simulink model "MPC_P2_2026_1"  (R2024b)
settings: Solver=VariableStepAuto  StartTime=0.0  StopTime=20  RelTol=1e-3
settings Model: Creator=Asus  LastModifiedBy=CARLOS
settings ModelReferenceCC: UpdateModelReferenceTargets=IfOutOfDate

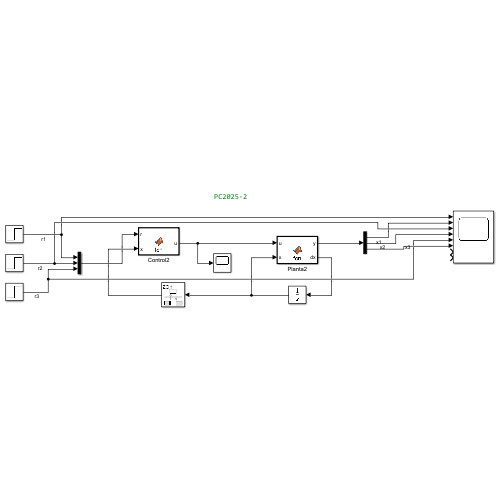
[thumbnail: Simulink's stored preview of the top-level diagram]
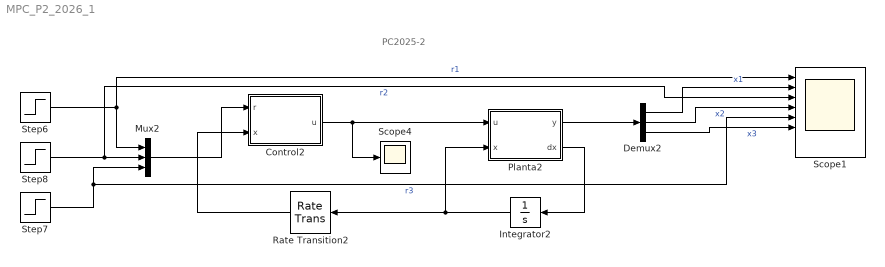
== system MPC_P2_2026_1 ==
  note: PC2025-2
  Control2 : MATLAB Function  TreatAsAtomicUnit=on
  Demux2 : Demux  Outputs=3
  Integrator2 : Integrator  InitialCondition=[0; 0; 0]
  Mux2 : Mux  Inputs=3
  Planta2 : MATLAB Function  TreatAsAtomicUnit=on
  Rate Transition2 : RateTransition  OutPortSampleTime=T
  Scope1 : Scope  NumInputPorts=8
  Scope4 : Scope
  Step6 : Step  After=0  SampleTime=0
  Step7 : Step  SampleTime=0
  Step8 : Step  After=0  SampleTime=0
  wires:
  Rate Transition2/1 -> Control2/2(x)
  Integrator2/1 -> Planta2/2(x), Rate Transition2/1
  Demux2/1 -> Scope1/2  "x1"
  Demux2/3 -> Scope1/6  "x3"
  Demux2/2 -> Scope1/4  "x2"
  Step7/1 -> Scope1/5, Mux2/3  "r3"
  Step8/1 -> Scope1/3, Mux2/2  "r2"
  Planta2/1(y) -> Demux2/1
  Step6/1 -> Mux2/1, Scope1/1  "r1"
  Control2/1(u) -> Scope4/1, Planta2/1(u)
  Planta2/2(dx) -> Integrator2/1
  Mux2/1 -> Control2/1(r)

== matlab function MPC_P2_2026_1/Planta2 ==
  data: u input; y output; dx output; x input
function [y, dx] = fcn(u, x)

A=[-2 -1 0;
    0 -2 1;
    0 0 -2]
B = [1;0;3]
C = eye(3)
D = [0]

dx = A*x + B*u;
y = C*x + D*u;

== matlab function MPC_P2_2026_1/Control2 ==
  data: r input; u output; x input
function u = fcn(r, x)

Ad = [  0.8187	-0.0819	-0.0041;
0	0.8187	0.0819;
0	0	0.8187 ];
Bd = [ 0.0902;
0.0131;
0.2719];

% Horizonte de predicción
N = 4;

% Dimensiones del sistema
nx = 3; % número de estados
nu = 1; % número de entradas

Q = diag([1,1,100]);
R = 1;

u1max = 50;
x1max = 50;
x2max = 50;
x3max = pi;


% Matrices auxiliares
In = eye(nx);          % matriz identidad nx x nx
Zn = zeros(nx);        % matriz de ceros nx x nx
Zm = zeros(nx, nu);    % matriz de ceros nx x nu

% Construcción de la matriz H (término cuadrático del QP)
% blkdiag arma una matriz diagonal por bloques: [R 0 0; 0 R 0; 0 0 R; Q 0 0; 0 Q 0; 0 0 Q]
H = 2*blkdiag(R, R, R, R, Q, Q, Q, Q);

% Término lineal del QP (depende de la referencia)
% -2*[0;0;0;Q*r;Q*r;Q*r] penaliza la distancia del estado a la referencia en las 3 etapas
f = -2*[0; 0; 0; 0; Q*r; Q*r; Q*r; Q*r];

% Restricciones de desigualdad (vacías en este caso, no usas inecuaciones explícitas)
Ain = [];
bin = [];

% Restricciones de igualdad (dinámica del sistema)
% Cada fila impone: x(k+1) = Ad*x(k) + Bd*u(k)

Aeq = [-Bd, Zm, Zm, Zm, In, Zn, Zn, Zn;
       Zm, -Bd, Zm, Zm, -Ad, In, Zn, Zn;
       Zm, Zm, -Bd, Zm, Zn, -Ad, In, Zn;
       Zm, Zm, Zm, -Bd, Zn, Zn, -Ad, In;]

% Lado derecho de las ecuaciones (condiciones iniciales y zeros)
beq = [Ad*x; Zm; Zm; Zm];

% Bloque de Limites
lb_x = [-x1max; -x2max; -x3max];
ub_x = [ x1max;  x2max;  x3max];

% Límites inferiores (control y estados)
lb = [-u1max; -u1max; -u1max; -u1max; lb_x; lb_x; lb_x; lb_x];

% Límites superiores
ub = [u1max; u1max; u1max; u1max;ub_x; ub_x; ub_x; ub_x];

z0 = zeros(N*(nx+nu),1);
options = optimoptions('quadprog', 'Algorithm','active-set', 'Display', 'off')

z = quadprog(H,f,Ain,bin,Aeq,beq,lb,ub,z0,options)
u = z(1);
